simulink library "HEMERO"  (Simulink 3.00)
values from neighbouring files (symbols this model uses):
  K1 = 0.5    [ejh64.m]    (also in ejh65.m)
  K2 = 0.8    [ejh64.m]    (also in ejh65.m)
  x_camino = 0:0.01:10    [ejh64.m]    (also in ejh65.m)
  y_camino = x_camino.^2    [ejh64.m]    (also in ejh65.m)
undefined symbols (not defined in the file or in its folder): magnitude, nonlinear
libraries: simulink_extras x12, HEMERO x9, simulink3 x6, dspstat x4
(part 2 of 9)

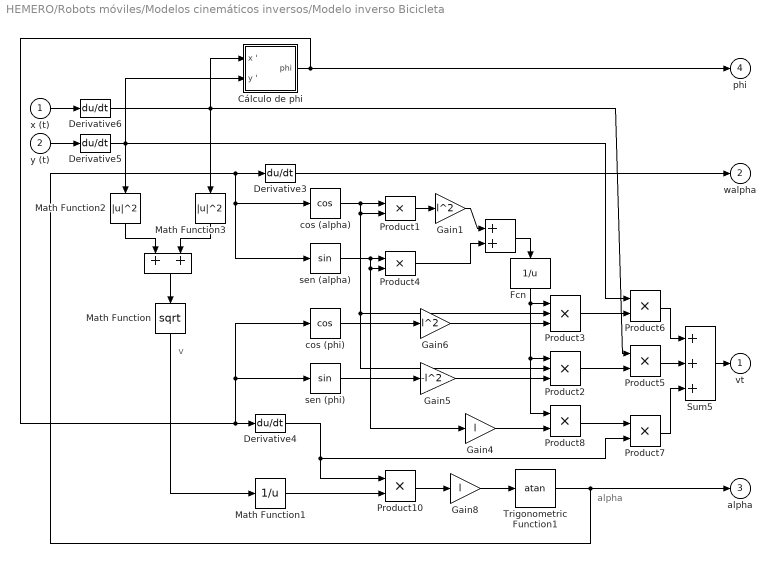
== system HEMERO/Robots móviles/Modelos cinemáticos inversos/Modelo inverso Bicicleta ==
  note: v
  note: alpha
  x (t) : Inport  Port=1  PortWidth=-1  SampleTime=-1  DataType=auto
      settings: SignalType=auto
  y (t) : Inport  Port=2  PortWidth=-1  SampleTime=-1  DataType=auto
      settings: SignalType=auto
  " " : Sum  Inputs=++  SaturateOnIntegerOverflow=on
  "  " : Sum  Orientation=down  Inputs=++  SaturateOnIntegerOverflow=on
  Cálculo de phi : Subsystem
  Derivative{3..6} (4 alike) : Derivative
  Fcn : Fcn  Orientation=down  Expr=1/u
  Gain1 : Gain  Gain=l^2  SaturateOnIntegerOverflow=on
  Gain4 : Gain  Gain=l  SaturateOnIntegerOverflow=on
  Gain5 : Gain  Gain=-l^2  SaturateOnIntegerOverflow=on
  Gain6 : Gain  Gain=l^2  SaturateOnIntegerOverflow=on
  Gain8 : Gain  Gain=l  SaturateOnIntegerOverflow=on
  Math Function : Math  Orientation=down  Operator=sqrt  OutputSignalType=auto
  Math Function1 : Math  Operator=reciprocal  OutputSignalType=auto
  Math Function2 : Math  Orientation=down  Operator=magnitude^2  OutputSignalType=auto
  Math Function3 : Math  Orientation=down  Operator=magnitude^2  OutputSignalType=auto
  Product{1,4..8,10} (7 alike) : Product  Inputs=2  SaturateOnIntegerOverflow=on
  Product2 : Product  Inputs=3  SaturateOnIntegerOverflow=on
  Product3 : Product  Inputs=3  SaturateOnIntegerOverflow=on
  Sum5 : Sum  Inputs=+++  SaturateOnIntegerOverflow=on
  Trigonometric Function1 : Trigonometry  Operator=atan  OutputSignalType=auto
  cos (alpha) : Trigonometry  Operator=cos  OutputSignalType=auto
  cos (phi) : Trigonometry  Operator=cos  OutputSignalType=auto
  sen (alpha) : Trigonometry  Operator=sin  OutputSignalType=auto
  sen (phi) : Trigonometry  Operator=sin  OutputSignalType=auto
  vt : Outport  Port=1  InitialOutput=0
  walpha : Outport  Port=2  InitialOutput=0
  alpha : Outport  Port=3  InitialOutput=0
  phi : Outport  Port=4  InitialOutput=0
  wires:
  Trigonometric Function1/1 -> alpha/1, Derivative3/1, cos (alpha)/1, sen (alpha)/1
  Cálculo de phi/1(phi) -> phi/1, cos (phi)/1, sen (phi)/1, Derivative4/1
  Math Function/1 -> Math Function1/1
  x (t)/1 -> Derivative6/1
  y (t)/1 -> Derivative5/1
  "  "/1 -> Math Function/1
  Math Function2/1 -> "  "/1
  Math Function3/1 -> "  "/2
  Derivative6/1 -> Math Function3/1, Product5/1, Cálculo de phi/1(x ')
  Derivative5/1 -> Math Function2/1, Product6/1, Cálculo de phi/2(y ')
  Gain8/1 -> Trigonometric Function1/1
  Product10/1 -> Gain8/1
  Math Function1/1 -> Product10/2
  Derivative4/1 -> Product10/1, Product7/2
  Product7/1 -> Sum5/3
  Product6/1 -> Sum5/1
  Product5/1 -> Sum5/2
  Derivative3/1 -> walpha/1
  Product8/1 -> Product7/1
  Sum5/1 -> vt/1
  Fcn/1 -> Product8/1, Product2/1, Product3/1
  Product2/1 -> Product5/2
  Gain6/1 -> Product3/3
  cos (phi)/1 -> Gain6/1
  Gain5/1 -> Product2/3
  sen (phi)/1 -> Gain5/1
  Product4/1 -> " "/2
  Product1/1 -> Gain1/1
  cos (alpha)/1 -> Product1/1, Product1/2, Product3/2, Product2/2
  sen (alpha)/1 -> Product4/2, Gain4/1, Product4/1
  " "/1 -> Fcn/1
  Gain1/1 -> " "/1
  Product3/1 -> Product6/2
  Gain4/1 -> Product8/2

== system HEMERO/Robots móviles/Modelos cinemáticos inversos/Modelo inverso Config. Síncrona ==
  x (t) : Inport  Port=1  PortWidth=-1  SampleTime=-1  DataType=auto
      settings: SignalType=auto
  y (t) : Inport  Port=2  PortWidth=-1  SampleTime=-1  DataType=auto
      settings: SignalType=auto
  Cálculo de phi : Subsystem
  Derivative : Derivative
  Derivative1 : Derivative
  Derivative2 : Derivative
  Product : Product  Inputs=2  SaturateOnIntegerOverflow=on
  Product1 : Product  Inputs=2  SaturateOnIntegerOverflow=on
  Sum : Sum  Inputs=-+  SaturateOnIntegerOverflow=on
  cos(phi) : Trigonometry  Operator=cos  OutputSignalType=auto
  sen(phi) : Trigonometry  Operator=sin  OutputSignalType=auto
  v : Outport  Port=1  InitialOutput=0
  w : Outport  Port=2  InitialOutput=0
  phi : Outport  Port=3  InitialOutput=0
  wires:
  Cálculo de phi/1(phi) -> phi/1, cos(phi)/1, Derivative2/1, sen(phi)/1
  Derivative1/1 -> Cálculo de phi/2(y '), Product1/1
  Derivative/1 -> Cálculo de phi/1(x '), Product/1
  cos(phi)/1 -> Product1/2
  sen(phi)/1 -> Product/2
  y (t)/1 -> Derivative1/1
  x (t)/1 -> Derivative/1
  Sum/1 -> v/1
  Product/1 -> Sum/1
  Product1/1 -> Sum/2
  Derivative2/1 -> w/1

== system HEMERO/Robots móviles/Modelos cinemáticos inversos/Modelo inverso Guiado Diferencial ==
  x (t) : Inport  Port=1  PortWidth=-1  SampleTime=-1  DataType=auto
      settings: SignalType=auto
  y (t) : Inport  Port=2  PortWidth=-1  SampleTime=-1  DataType=auto
      settings: SignalType=auto
  Cálculo de phi : Subsystem
  Derivative : Derivative
  Derivative1 : Derivative
  Derivative2 : Derivative
  Gain : Gain  Gain=b/2  SaturateOnIntegerOverflow=on
  Gain1 : Gain  Gain=1/c  SaturateOnIntegerOverflow=on
  Gain2 : Gain  Gain=1/c  SaturateOnIntegerOverflow=on
  Product : Product  Inputs=2  SaturateOnIntegerOverflow=on
  Product1 : Product  Inputs=2  SaturateOnIntegerOverflow=on
  Sum : Sum  Inputs=-+-  SaturateOnIntegerOverflow=on
  Sum1 : Sum  Inputs=-++  SaturateOnIntegerOverflow=on
  cos(phi) : Trigonometry  Operator=cos  OutputSignalType=auto
  sen(phi) : Trigonometry  Operator=sin  OutputSignalType=auto
  wi : Outport  Port=1  InitialOutput=0
  wd : Outport  Port=2  InitialOutput=0
  phi : Outport  Port=3  InitialOutput=0
  wires:
  x (t)/1 -> Derivative/1
  y (t)/1 -> Derivative1/1
  sen(phi)/1 -> Product/2
  cos(phi)/1 -> Product1/2
  Derivative2/1 -> Gain/1
  Product/1 -> Sum/1, Sum1/1
  Product1/1 -> Sum/2, Sum1/2
  Gain/1 -> Sum/3, Sum1/3
  Sum/1 -> Gain1/1
  Sum1/1 -> Gain2/1
  Derivative/1 -> Product/1, Cálculo de phi/1(x ')
  Derivative1/1 -> Product1/1, Cálculo de phi/2(y ')
  Cálculo de phi/1(phi) -> sen(phi)/1, Derivative2/1, cos(phi)/1, phi/1
  Gain1/1 -> wi/1
  Gain2/1 -> wd/1

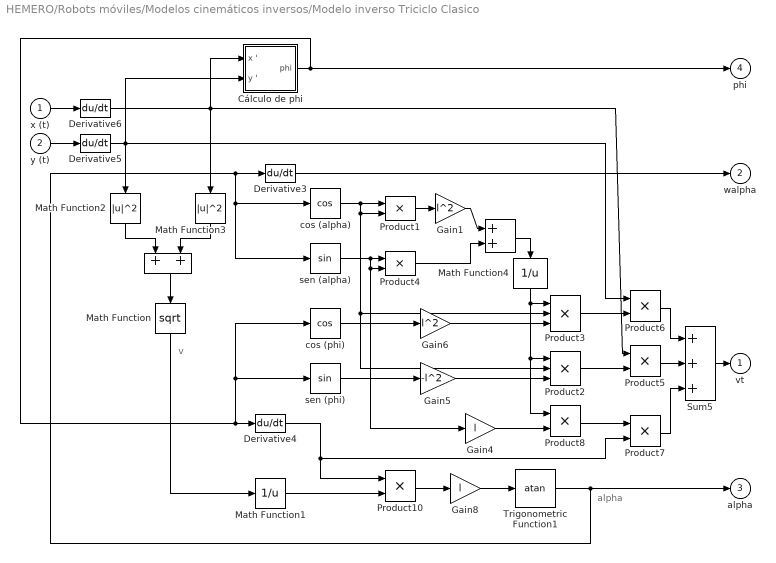
== system HEMERO/Robots móviles/Modelos cinemáticos inversos/Modelo inverso Triciclo Clasico ==
  note: alpha
  note: v
  x (t) : Inport  Port=1  PortWidth=-1  SampleTime=-1  DataType=auto
      settings: SignalType=auto
  y (t) : Inport  Port=2  PortWidth=-1  SampleTime=-1  DataType=auto
      settings: SignalType=auto
  " " : Sum  Inputs=++  SaturateOnIntegerOverflow=on
  "  " : Sum  Orientation=down  Inputs=++  SaturateOnIntegerOverflow=on
  Cálculo de phi : Subsystem
  Derivative{3..6} (4 alike) : Derivative
  Gain1 : Gain  Gain=l^2  SaturateOnIntegerOverflow=on
  Gain4 : Gain  Gain=l  SaturateOnIntegerOverflow=on
  Gain5 : Gain  Gain=-l^2  SaturateOnIntegerOverflow=on
  Gain6 : Gain  Gain=l^2  SaturateOnIntegerOverflow=on
  Gain8 : Gain  Gain=l  SaturateOnIntegerOverflow=on
  Math Function : Math  Orientation=down  Operator=sqrt  OutputSignalType=auto
  Math Function1 : Math  Operator=reciprocal  OutputSignalType=auto
  Math Function2 : Math  Orientation=down  Operator=magnitude^2  OutputSignalType=auto
  Math Function3 : Math  Orientation=down  Operator=magnitude^2  OutputSignalType=auto
  Math Function4 : Math  Orientation=down  Operator=reciprocal  OutputSignalType=auto
  Product{1,4..8,10} (7 alike) : Product  Inputs=2  SaturateOnIntegerOverflow=on
  Product2 : Product  Inputs=3  SaturateOnIntegerOverflow=on
  Product3 : Product  Inputs=3  SaturateOnIntegerOverflow=on
  Sum5 : Sum  Inputs=+++  SaturateOnIntegerOverflow=on
  Trigonometric Function1 : Trigonometry  Operator=atan  OutputSignalType=auto
  cos (alpha) : Trigonometry  Operator=cos  OutputSignalType=auto
  cos (phi) : Trigonometry  Operator=cos  OutputSignalType=auto
  sen (alpha) : Trigonometry  Operator=sin  OutputSignalType=auto
  sen (phi) : Trigonometry  Operator=sin  OutputSignalType=auto
  vt : Outport  Port=1  InitialOutput=0
  walpha : Outport  Port=2  InitialOutput=0
  alpha : Outport  Port=3  InitialOutput=0
  phi : Outport  Port=4  InitialOutput=0
  wires:
  Gain4/1 -> Product8/2
  Product3/1 -> Product6/2
  Gain1/1 -> " "/1
  " "/1 -> Math Function4/1
  sen (alpha)/1 -> Product4/1, Gain4/1, Product4/2
  cos (alpha)/1 -> Product2/2, Product3/2, Product1/2, Product1/1
  Product1/1 -> Gain1/1
  Product4/1 -> " "/2
  sen (phi)/1 -> Gain5/1
  Gain5/1 -> Product2/3
  cos (phi)/1 -> Gain6/1
  Gain6/1 -> Product3/3
  Product2/1 -> Product5/2
  Math Function4/1 -> Product3/1, Product2/1, Product8/1
  Sum5/1 -> vt/1
  Product8/1 -> Product7/1
  Derivative3/1 -> walpha/1
  Product5/1 -> Sum5/2
  Product6/1 -> Sum5/1
  Product7/1 -> Sum5/3
  Derivative4/1 -> Product7/2, Product10/1
  Math Function1/1 -> Product10/2
  Product10/1 -> Gain8/1
  Gain8/1 -> Trigonometric Function1/1
  Derivative5/1 -> Cálculo de phi/2(y '), Product6/1, Math Function2/1
  Derivative6/1 -> Cálculo de phi/1(x '), Product5/1, Math Function3/1
  Math Function3/1 -> "  "/2
  Math Function2/1 -> "  "/1
  "  "/1 -> Math Function/1
  y (t)/1 -> Derivative5/1
  x (t)/1 -> Derivative6/1
  Math Function/1 -> Math Function1/1
  Cálculo de phi/1(phi) -> Derivative4/1, sen (phi)/1, cos (phi)/1, phi/1
  Trigonometric Function1/1 -> sen (alpha)/1, cos (alpha)/1, Derivative3/1, alpha/1

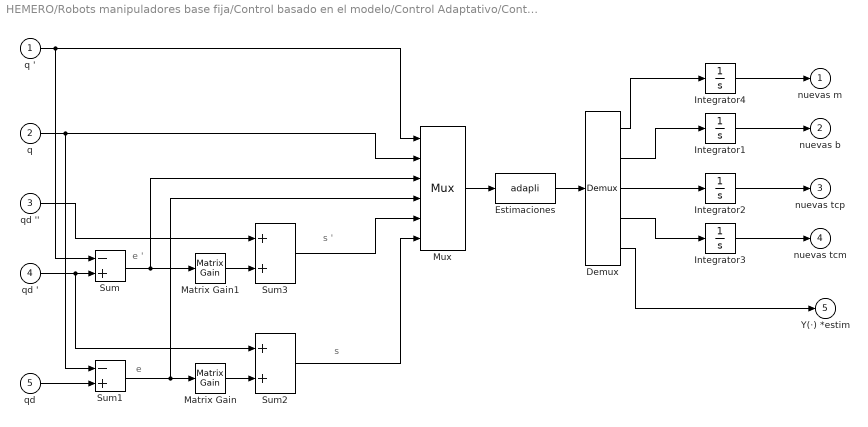
== system HEMERO/Robots manipuladores base fija/Control basado en el modelo/Control Adaptativo/Control de inercia adaptativo ==
  note: e
  note: e '
  note: s
  note: s '
  q ' : Inport  Port=1  PortWidth=-1  SampleTime=-1  DataType=auto
      settings: SignalType=auto
  q : Inport  Port=2  PortWidth=-1  SampleTime=-1  DataType=auto
      settings: SignalType=auto
  qd '' : Inport  Port=3  PortWidth=-1  SampleTime=-1  DataType=auto
      settings: SignalType=auto
  qd ' : Inport  Port=4  PortWidth=-1  SampleTime=-1  DataType=auto
      settings: SignalType=auto
  qd : Inport  Port=5  PortWidth=-1  SampleTime=-1  DataType=auto
      settings: SignalType=auto
  Demux : Demux  Outputs=5
  Estimaciones : S-Function  FunctionName=adapli  Parameters=dyn, gamma, a, grav  PortCounts=[]  SFunctionModules=''
  Integrator1 : Integrator  ExternalReset=none  InitialConditionSource=internal  InitialCondition=b_inicial(:)  LimitOutput=off  UpperSaturationLimit=inf  LowerSaturationLimit=-inf  ShowSaturationPort=off  ShowStatePort=off  AbsoluteTolerance=auto
  Integrator2 : Integrator  ExternalReset=none  InitialConditionSource=internal  InitialCondition=tcp_inicial(:)  LimitOutput=off  UpperSaturationLimit=inf  LowerSaturationLimit=-inf  ShowSaturationPort=off  ShowStatePort=off  AbsoluteTolerance=auto
  Integrator3 : Integrator  ExternalReset=none  InitialConditionSource=internal  InitialCondition=tcm_inicial(:)  LimitOutput=off  UpperSaturationLimit=inf  LowerSaturationLimit=-inf  ShowSaturationPort=off  ShowStatePort=off  AbsoluteTolerance=auto
  Integrator4 : Integrator  ExternalReset=none  InitialConditionSource=internal  InitialCondition=m_inicial(:)  LimitOutput=off  UpperSaturationLimit=inf  LowerSaturationLimit=-inf  ShowSaturationPort=off  ShowStatePort=off  AbsoluteTolerance=auto
  Matrix Gain : simulink3/Math/Matrix Gain  K=a
  Matrix Gain1 : simulink3/Math/Matrix Gain  K=a
  Mux : Mux  Inputs=6
      settings: DisplayOption=none
  Sum : Sum  Inputs=-+  SaturateOnIntegerOverflow=on
  Sum1 : Sum  Inputs=-+  SaturateOnIntegerOverflow=on
  Sum2 : Sum  Inputs=++  SaturateOnIntegerOverflow=on
  Sum3 : Sum  Inputs=++  SaturateOnIntegerOverflow=on
  nuevas m : Outport  Port=1  InitialOutput=0
  nuevas b : Outport  Port=2  InitialOutput=0
  nuevas tcp : Outport  Port=3  InitialOutput=0
  nuevas tcm : Outport  Port=4  InitialOutput=0
  Y(·) *estim : Outport  Port=5  InitialOutput=0
  wires:
  q '/1 -> Mux/1, Sum/1
  q/1 -> Mux/2, Sum1/1
  Mux/1 -> Estimaciones/1
  Estimaciones/1 -> Demux/1
  Demux/2 -> Integrator1/1
  Integrator1/1 -> nuevas b/1
  Demux/3 -> Integrator2/1
  Integrator2/1 -> nuevas tcp/1
  Demux/4 -> Integrator3/1
  Integrator3/1 -> nuevas tcm/1
  qd/1 -> Sum1/2
  Matrix Gain/1 -> Sum2/2
  qd '/1 -> Sum/2, Sum2/1
  Matrix Gain1/1 -> Sum3/2
  qd ''/1 -> Sum3/1
  Sum2/1 -> Mux/6
  Sum3/1 -> Mux/5
  Sum/1 -> Matrix Gain1/1, Mux/3
  Sum1/1 -> Matrix Gain/1, Mux/4
  Demux/5 -> Y(·) *estim/1
  Demux/1 -> Integrator4/1
  Integrator4/1 -> nuevas m/1

== system HEMERO/Robots manipuladores base fija/Control basado en el modelo/Control Adaptativo/Ejemplos ==
  Ejemplo H.5.5 : Subsystem

== system HEMERO/Robots manipuladores base fija/Control basado en el modelo/Control Adaptativo/Inversa de la matriz de masas ==
  q : Inport  Port=1  PortWidth=-1  SampleTime=-1  DataType=auto
      settings: SignalType=auto
  In : Inport  Port=2  PortWidth=-1  SampleTime=-1  DataType=auto
      settings: SignalType=auto
  nuevas m : Inport  Port=3  PortWidth=-1  SampleTime=-1  DataType=auto
      settings: SignalType=auto
  Masas : S-Function  FunctionName=esminv  Parameters=dyn  PortCounts=[]  SFunctionModules=''
  Mux : Mux  Inputs=3
      settings: DisplayOption=none
  M(q)^(-1) · In : Outport  Port=1  InitialOutput=0
  wires:
  q/1 -> Mux/1
  In/1 -> Mux/2
  nuevas m/1 -> Mux/3
  Mux/1 -> Masas/1
  Masas/1 -> M(q)^(-1) · In/1

== system HEMERO/Robots manipuladores base fija/Control basado en el modelo/Control Adaptativo/Modelo de fricciones ==
  q' : Inport  Port=1  PortWidth=-1  SampleTime=-1  DataType=auto
      settings: SignalType=auto
  nuevas b : Inport  Port=2  PortWidth=-1  SampleTime=-1  DataType=auto
      settings: SignalType=auto
  nuevas tcp : Inport  Port=3  PortWidth=-1  SampleTime=-1  DataType=auto
      settings: SignalType=auto
  nuevas tcm : Inport  Port=4  PortWidth=-1  SampleTime=-1  DataType=auto
      settings: SignalType=auto
  Fricciones : S-Function  FunctionName=esfriction  Parameters=G,b,tcp,tcm  PortCounts=[]  SFunctionModules=''
  Mux : Mux  Inputs=4
      settings: DisplayOption=none
  tau_f : Outport  Port=1  InitialOutput=0
  wires:
  Mux/1 -> Fricciones/1
  q'/1 -> Mux/1
  nuevas b/1 -> Mux/2
  nuevas tcp/1 -> Mux/3
  nuevas tcm/1 -> Mux/4
  Fricciones/1 -> tau_f/1

== system HEMERO/Robots manipuladores base fija/Control basado en el modelo/Control Adaptativo/Término Vm de Coriolis ==
  q : Inport  Port=1  PortWidth=-1  SampleTime=-1  DataType=auto
      settings: SignalType=auto
  q ' : Inport  Port=2  PortWidth=-1  SampleTime=-1  DataType=auto
      settings: SignalType=auto
  In : Inport  Port=3  PortWidth=-1  SampleTime=-1  DataType=auto
      settings: SignalType=auto
  nuevas m : Inport  Port=4  PortWidth=-1  SampleTime=-1  DataType=auto
      settings: SignalType=auto
  "  " : S-Function  FunctionName=esvmcorioli  Parameters=dyn  PortCounts=[]  SFunctionModules=''
  Mux : Mux  Inputs=4
      settings: DisplayOption=none
  Vm (q,q')·In : Outport  Port=1  InitialOutput=0
  wires:
  q '/1 -> Mux/2
  q/1 -> Mux/1
  In/1 -> Mux/3
  Mux/1 -> "  "/1
  "  "/1 -> Vm (q,q')·In/1
  nuevas m/1 -> Mux/4

== system HEMERO/Robots manipuladores base fija/Control basado en el modelo/Control Adaptativo/Término de la matriz de masas ==
  q : Inport  Port=1  PortWidth=-1  SampleTime=-1  DataType=auto
      settings: SignalType=auto
  In : Inport  Port=2  PortWidth=-1  SampleTime=-1  DataType=auto
      settings: SignalType=auto
  nuevas m : Inport  Port=3  PortWidth=-1  SampleTime=-1  DataType=auto
      settings: SignalType=auto
  Masas : S-Function  FunctionName=esinertia  Parameters=dyn  PortCounts=[]  SFunctionModules=''
  Mux : Mux  Inputs=3
      settings: DisplayOption=none
  M (q)·In : Outport  Port=1  InitialOutput=0
  wires:
  In/1 -> Mux/2
  q/1 -> Mux/1
  Mux/1 -> Masas/1
  Masas/1 -> M (q)·In/1
  nuevas m/1 -> Mux/3

== system HEMERO/Robots manipuladores base fija/Control basado en el modelo/Control Adaptativo/Términos gravitatorios ==
  q : Inport  Port=1  PortWidth=-1  SampleTime=-1  DataType=auto
      settings: SignalType=auto
  nuevas m : Inport  Port=2  PortWidth=-1  SampleTime=-1  DataType=auto
      settings: SignalType=auto
  Gravedad : S-Function  FunctionName=esgravity  Parameters=dyn,grav  PortCounts=[]  SFunctionModules=''
  Mux : Mux  Inputs=2
      settings: DisplayOption=none
  G (q) : Outport  Port=1  InitialOutput=0
  wires:
  Gravedad/1 -> G (q)/1
  q/1 -> Mux/1
  nuevas m/1 -> Mux/2
  Mux/1 -> Gravedad/1

== system HEMERO/Robots manipuladores base fija/Control basado en el modelo/Control Adaptativo/Términos centrífugos y de Coriolis ==
  q : Inport  Port=1  PortWidth=-1  SampleTime=-1  DataType=auto
      settings: SignalType=auto
  q' : Inport  Port=2  PortWidth=-1  SampleTime=-1  DataType=auto
      settings: SignalType=auto
  nuevas m : Inport  Port=3  PortWidth=-1  SampleTime=-1  DataType=auto
      settings: SignalType=auto
  Centrífugos y Coriolis : S-Function  FunctionName=escoriolis  Parameters=dyn  PortCounts=[]  SFunctionModules=''
  Mux : Mux  Inputs=3
      settings: DisplayOption=none
  V (q,q') : Outport  Port=1  InitialOutput=0
  wires:
  nuevas m/1 -> Mux/3
  Mux/1 -> Centrífugos y Coriolis/1
  Centrífugos y Coriolis/1 -> V (q,q')/1
  q/1 -> Mux/1
  q'/1 -> Mux/2

== system HEMERO/Robots manipuladores base fija/Control basado en el modelo/Control con aprendizaje/Ejemplos ==
  Ejemplo H.5.1 : Subsystem

== system HEMERO/Robots manipuladores base fija/Control basado en el modelo/Control con aprendizaje/Par realimentado aprendido ==
  note: e ''
  note: e '
  note: e
  qd '' : Inport  Port=1  PortWidth=-1  SampleTime=-1  DataType=auto
      settings: SignalType=auto
  q '' : Inport  Port=2  PortWidth=-1  SampleTime=-1  DataType=auto
      settings: SignalType=auto
  qd ' : Inport  Port=3  PortWidth=-1  SampleTime=-1  DataType=auto
      settings: SignalType=auto
  q ' : Inport  Port=4  PortWidth=-1  SampleTime=-1  DataType=auto
      settings: SignalType=auto
  qd : Inport  Port=5  PortWidth=-1  SampleTime=-1  DataType=auto
      settings: SignalType=auto
  q : Inport  Port=6  PortWidth=-1  SampleTime=-1  DataType=auto
      settings: SignalType=auto
  Demux : Demux  Outputs=4
  Mux : Mux  Inputs=3
      settings: DisplayOption=none
  S-Function : S-Function  FunctionName=learn  Parameters=Kp, Kv, mu, tfinal  PortCounts=[]  SFunctionModules=''
  Sum : Sum  Inputs=+-  SaturateOnIntegerOverflow=on
  Sum1 : Sum  Inputs=+-  SaturateOnIntegerOverflow=on
  Sum2 : Sum  Inputs=+-  SaturateOnIntegerOverflow=on
  To Workspace1 : ToWorkspace  VariableName=error  SampleTime=-1  SaveFormat=Matrix
  To Workspace2 : ToWorkspace  VariableName=error_d  SampleTime=-1  SaveFormat=Matrix
  To Workspace3 : ToWorkspace  VariableName=error_dd  SampleTime=-1  SaveFormat=Matrix
  To Workspace4 : ToWorkspace  VariableName=edd  SampleTime=-1  SaveFormat=Matrix
  To Workspace5 : ToWorkspace  VariableName=dknueva  SampleTime=-1  SaveFormat=Matrix
  To Workspace6 : ToWorkspace  VariableName=ed  SampleTime=-1  SaveFormat=Matrix
  To Workspace7 : ToWorkspace  VariableName=e  SampleTime=-1  SaveFormat=Matrix
  Término de la matriz de masas estimado : Subsystem  mask(Término asociado a la matriz de masas){dyn=dyn}
      mask prompts: dyn "Matriz de parámetros cinemáticos y dinámicos:"
      mask help: Este bloque calcula el par correspondiente al término en el que aparece la matriz de masas.
  gamma (k) : Outport  Port=1
  wires:
  Mux/1 -> S-Function/1
  S-Function/1 -> Demux/1
  qd ''/1 -> Sum/1
  q ''/1 -> Sum/2
  qd '/1 -> Sum1/1
  q '/1 -> Sum1/2
  qd/1 -> Sum2/1
  Demux/1 -> Término de la matriz de masas estimado/2(In), To Workspace5/1
  Sum2/1 -> Mux/3, To Workspace7/1
  Sum1/1 -> Mux/2, To Workspace6/1
  Sum/1 -> Mux/1, To Workspace4/1
  Demux/2 -> To Workspace1/1
  Demux/3 -> To Workspace2/1
  Demux/4 -> To Workspace3/1
  q/1 -> Sum2/2, Término de la matriz de masas estimado/1(q)
  Término de la matriz de masas estimado/1(M (q)·In) -> gamma (k)/1

== system HEMERO/Robots manipuladores base fija/Control basado en el modelo/Par Computado/Control PD ==
  qd : Inport  Port=1  PortWidth=-1  SampleTime=-1  DataType=auto
      settings: SignalType=auto
  q : Inport  Port=2  PortWidth=-1  SampleTime=-1  DataType=auto
      settings: SignalType=auto
  qd' : Inport  Port=3  PortWidth=-1  SampleTime=-1  DataType=auto
      settings: SignalType=auto
  q' : Inport  Port=4  PortWidth=-1  SampleTime=-1  DataType=auto
      settings: SignalType=auto
  qd'' : Inport  Port=5  PortWidth=-1  SampleTime=-1  DataType=auto
      settings: SignalType=auto
  Kp : StateSpace  A=[]  B=[]  C=[]  D=K  X0=0  mask(Matrix Gain){@1=Kp}
      mask prompts: @1 "Gain matrix:"
      mask help: Matrix Gain.
      mask init:
      | K=@1;
      mask Help: Multiplies input vector by entered matrix to produce output vector (y=Au).
      mask Display: disp('K')
  Kv : StateSpace  A=[]  B=[]  C=[]  D=K  X0=0  mask(Matrix Gain){@1=Kv}
      mask prompts: @1 "Gain matrix:"
      mask help: Matrix Gain.
      mask init:
      | K=@1;
      mask Help: Multiplies input vector by entered matrix to produce output vector (y=Au).
      mask Display: disp('K')
  Sum : Sum  Inputs=+-  SaturateOnIntegerOverflow=on
  Sum1 : Sum  Inputs=+-  SaturateOnIntegerOverflow=on
  Sum2 : Sum  Inputs=+++  SaturateOnIntegerOverflow=on
  tau_r : Outport  Port=1  InitialOutput=0
  wires:
  Sum2/1 -> tau_r/1
  qd''/1 -> Sum2/3
  Kp/1 -> Sum2/1
  Kv/1 -> Sum2/2
  Sum1/1 -> Kv/1
  Sum/1 -> Kp/1
  q'/1 -> Sum1/2
  qd'/1 -> Sum1/1
  q/1 -> Sum/2
  qd/1 -> Sum/1

== system HEMERO/Robots manipuladores base fija/Control basado en el modelo/Par Computado/Control PID ==
  note: e
  note: e'
  qd : Inport  Port=1  PortWidth=-1  SampleTime=-1  DataType=auto
      settings: SignalType=auto
  q : Inport  Port=2  PortWidth=-1  SampleTime=-1  DataType=auto
      settings: SignalType=auto
  qd' : Inport  Port=3  PortWidth=-1  SampleTime=-1  DataType=auto
      settings: SignalType=auto
  q' : Inport  Port=4  PortWidth=-1  SampleTime=-1  DataType=auto
      settings: SignalType=auto
  qd'' : Inport  Port=5  PortWidth=-1  SampleTime=-1  DataType=auto
      settings: SignalType=auto
  Integrator : Integrator  ExternalReset=none  InitialConditionSource=internal  InitialCondition=0  LimitOutput=off  UpperSaturationLimit=inf  LowerSaturationLimit=-inf  ShowSaturationPort=off  ShowStatePort=off  AbsoluteTolerance=auto
  Ki : StateSpace  A=[]  B=[]  C=[]  D=K  X0=0  mask(Matrix Gain){@1=Ki}
      mask prompts: @1 "Gain matrix:"
      mask help: Matrix Gain.
      mask init:
      | K=@1;
      mask Help: Multiplies input vector by entered matrix to produce output vector (y=Au).
      mask Display: disp('K')
  Kp : StateSpace  A=[]  B=[]  C=[]  D=K  X0=0  mask(Matrix Gain){@1=Kp}
      mask prompts: @1 "Gain matrix:"
      mask help: Matrix Gain.
      mask init:
      | K=@1;
      mask Help: Multiplies input vector by entered matrix to produce output vector (y=Au).
      mask Display: disp('K')
  Kv : StateSpace  A=[]  B=[]  C=[]  D=K  X0=0  mask(Matrix Gain){@1=Kv}
      mask prompts: @1 "Gain matrix:"
      mask help: Matrix Gain.
      mask init:
      | K=@1;
      mask Help: Multiplies input vector by entered matrix to produce output vector (y=Au).
      mask Display: disp('K')
  Sum : Sum  Inputs=+-  SaturateOnIntegerOverflow=on
  Sum1 : Sum  Inputs=+-  SaturateOnIntegerOverflow=on
  Sum2 : Sum  Inputs=++++  SaturateOnIntegerOverflow=on
  tau_r : Outport  Port=1  InitialOutput=0
  wires:
  Sum2/1 -> tau_r/1
  Sum1/1 -> Kv/1
  q'/1 -> Sum1/2
  qd'/1 -> Sum1/1
  q/1 -> Sum/2
  qd/1 -> Sum/1
  qd''/1 -> Sum2/4
  Kv/1 -> Sum2/3
  Kp/1 -> Sum2/2
  Sum/1 -> Kp/1, Ki/1
  Ki/1 -> Integrator/1
  Integrator/1 -> Sum2/1

== system HEMERO/Robots manipuladores base fija/Control basado en el modelo/Par Computado/Ejemplos ==
  Ejemplo H.5.2 : Subsystem
  Ejemplo H.5.3 : Subsystem
  Ejemplo H.5.4 : Subsystem

== system HEMERO/Robots manipuladores base fija/Modelo Dinámico/Ejemplos/Ejemplo H.4.2 ==
  Mux : Mux  Inputs=2
      settings: DisplayOption=none
  Tiempo : Clock
      settings: DisplayTime=off  Decimation=10
  To Workspace1 : ToWorkspace  VariableName=q  SampleTime=-1  SaveFormat=Matrix
  Trayectorias articulares : Subsystem  mask(Trayectorias articulares){dyn=[0 0 0 0 0 2 3 0 0 0 0 0 0 0 0 0 1 0 0 0; 0 3 0 0 0 1 1 0 0 0 0 0 0 0 0 0 1 0 0 0], grav=[0 -9.81 0], inivel=[0 0], inipos=[0 0]}
      mask prompts: dyn "Matriz de parámetros cinemáticos y dinámicos:"; grav "Vector aceleración de la gravedad:"; inivel "Velocidades articulares iniciales:"; inipos "Posiciones articulares iniciales:"
      mask help: Se calculan las trayectorias articulares (posiciones, velocidades y aceleraciones articulares) a partir de los pares aplicados al manipulador.
  tau1 : Fcn  Expr=30+(1+exp(-u))*10*sin(u)
  tau2 : Fcn  Expr=10+10*cos(u)
  wires:
  Mux/1 -> Trayectorias articulares/1(tau)
  Trayectorias articulares/1(q) -> To Workspace1/1
  Tiempo/1 -> tau1/1, tau2/1
  tau1/1 -> Mux/1
  tau2/1 -> Mux/2

== system HEMERO/Robots manipuladores base fija/Modelo Dinámico/Ejemplos/Ejemplo H.4.4a ==
  note: q'
  note: q''
  note: q
  Integrator : Integrator  ExternalReset=none  InitialConditionSource=internal  InitialCondition=[0;0;0]  LimitOutput=off  UpperSaturationLimit=inf  LowerSaturationLimit=-inf  ShowSaturationPort=off  ShowStatePort=off  AbsoluteTolerance=auto
  Integrator1 : Integrator  ExternalReset=none  InitialConditionSource=internal  InitialCondition=[-pi/2; 0; 0]  LimitOutput=off  UpperSaturationLimit=inf  LowerSaturationLimit=-inf  ShowSaturationPort=off  ShowStatePort=off  AbsoluteTolerance=auto
  Inversa de la matriz de masas : Subsystem  mask(Término de Coriolis){dyn=[0 0 0 0 0 4.7 0.8 0 0 0 0 0 0 0 0 0 1 0 0 0;0 0.8 0 0 0 2.6 0.8 0 0 0 0 0 0 0 0 0 1 0 0 0;0 0.8 0 0 0 1.1 0 0 0 0.05 0.1 0.1 0 0 0 0 1 0 0 0]}
      mask prompts: dyn "Matriz de parámetros dinámicos:"
      mask help: Este bloque devuelve el par correspondiente al término de Coriolis.
      mask Help: A este bloque hay que darle tres parámetros: 1) La matriz de parámetros dinámicos del manipulador de acuerdo con el formato que se explica en la sección "dyn" del Apéndice, 2) Un vector columna correspondiente a la aceleración de la gravedad, y 3) Un vector columna correspondiente a las fuerzas externas.
  Sum : Sum  Inputs=+--  SaturateOnIntegerOverflow=on
  To Workspace : ToWorkspace  VariableName=q  SampleTime=-1  SaveFormat=Matrix
  Términos gravitatorios : Subsystem  mask(Término gravitatorio){dyn=[0 0 0 0 0 4.7 0.8 0 0 0 0 0 0 0 0 0 1 0 0 0;0 0.8 0 0 0 2.6 0.8 0 0 0 0 0 0 0 0 0 1 0 0 0;0 0.8 0 0 0 1.1 0 0 0 0.05 0.1 0.1 0 0 0 0 1 0 0 0], grav=[0 -9.8 0]}
      mask prompts: dyn "Matriz de parámetros cinemáticos y dinámicos:"; grav "Vector aceleración de la gravedad:"
      mask help: Este bloque calcula el par correspondiente al término gravitatorio.
  Términos centrífugos y de Coriolis : Subsystem  mask(Términos centrífugos y de Coriolis){dyn=[0 0 0 0 0 4.7 0.8 0 0 0 0 0 0 0 0 0 1 0 0 0;0 0.8 0 0 0 2.6 0.8 0 0 0 0 0 0 0 0 0 1 0 0 0;0 0.8 0 0 0 1.1 0 0 0 0.05 0.1 0.1 0 0 0 0 1 0 0 0]}
      mask prompts: dyn "Matriz de parámetros cinemáticos y dinámicos:"
      mask help: Este bloque calcula el par correspondiente a los términos centrífugos y de Coriolis.
  q : Display
      settings: Format=short
  tau : Constant  Value=[0;0;0]
  wires:
  Términos centrífugos y de Coriolis/1(V (q,q')) -> Sum/2
  Sum/1 -> Inversa de la matriz de masas/2(In)
  Inversa de la matriz de masas/1(M(q)^(-1) · In) -> Integrator/1
  Integrator/1 -> Integrator1/1, Términos centrífugos y de Coriolis/2(q')
  Integrator1/1 -> Inversa de la matriz de masas/1(q), To Workspace/1, Términos centrífugos y de Coriolis/1(q), Términos gravitatorios/1(q), q/1
  Términos gravitatorios/1(G (q)) -> Sum/3
  tau/1 -> Sum/1

== system HEMERO/Robots manipuladores base fija/Modelo Dinámico/Ejemplos/Ejemplo H.4.4b ==
  note: q'
  note: q''
  note: q
  Integrator : Integrator  ExternalReset=none  InitialConditionSource=internal  InitialCondition=[0;0;0]  LimitOutput=off  UpperSaturationLimit=inf  LowerSaturationLimit=-inf  ShowSaturationPort=off  ShowStatePort=off  AbsoluteTolerance=auto
  Integrator1 : Integrator  ExternalReset=none  InitialConditionSource=internal  InitialCondition=[pi/6; pi/6; pi/18]  LimitOutput=off  UpperSaturationLimit=inf  LowerSaturationLimit=-inf  ShowSaturationPort=off  ShowStatePort=off  AbsoluteTolerance=auto
  Inversa de la matriz de masas : Subsystem  mask(Término de Coriolis){dyn=[0 0 0 0 0 4.7 0.8 0 0 0 0 0 0 0 0 0 1 0 0 0;0 0.8 0 0 0 2.6 0.8 0 0 0 0 0 0 0 0 0 1 0 0 0;0 0.8 0 0 0 1.1 0 0 0 0.05 0.1 0.1 0 0 0 0 1 0 0 0]}
      mask prompts: dyn "Matriz de parámetros dinámicos:"
      mask help: Este bloque devuelve el par correspondiente al término de Coriolis.
      mask Help: A este bloque hay que darle tres parámetros: 1) La matriz de parámetros dinámicos del manipulador de acuerdo con el formato que se explica en la sección "dyn" del Apéndice, 2) Un vector columna correspondiente a la aceleración de la gravedad, y 3) Un vector columna correspondiente a las fuerzas externas.
  Sum : Sum  Inputs=+--  SaturateOnIntegerOverflow=on
  To Workspace : ToWorkspace  VariableName=q  SampleTime=-1  SaveFormat=Matrix
  Términos gravitatorios : Subsystem  mask(Término gravitatorio){dyn=[0 0 0 0 0 4.7 0.8 0 0 0 0 0 0 0 0 0 1 0 0 0;0 0.8 0 0 0 2.6 0.8 0 0 0 0 0 0 0 0 0 1 0 0 0;0 0.8 0 0 0 1.1 0 0 0 0.05 0.1 0.1 0 0 0 0 1 0 0 0], grav=[0 -9.8 0]}
      mask prompts: dyn "Matriz de parámetros cinemáticos y dinámicos:"; grav "Vector aceleración de la gravedad:"
      mask help: Este bloque calcula el par correspondiente al término gravitatorio.
  Términos centrífugos y de Coriolis : Subsystem  mask(Término de Coriolis){dyn=[0 0 0 0 0 4.7 0.8 0 0 0 0 0 0 0 0 0 1 0 0 0;0 0.8 0 0 0 2.6 0.8 0 0 0 0 0 0 0 0 0 1 0 0 0;0 0.8 0 0 0 1.1 0 0 0 0.05 0.1 0.1 0 0 0 0 1 0 0 0]}
      mask prompts: dyn "Matriz de parámetros dinámicos:"
      mask help: Este bloque devuelve el par correspondiente al término de Coriolis.
      mask Help: A este bloque hay que darle tres parámetros: 1) La matriz de parámetros dinámicos del manipulador de acuerdo con el formato que se explica en la sección "dyn" del Apéndice, 2) Un vector columna correspondiente a la aceleración de la gravedad, y 3) Un vector columna correspondiente a las fuerzas externas.
  q : Display
      settings: Format=short
  tau : Constant  Value=[0;0;0]
  wires:
  Términos centrífugos y de Coriolis/1(V (q,q')) -> Sum/2
  Sum/1 -> Inversa de la matriz de masas/2(In)
  Inversa de la matriz de masas/1(M(q)^(-1) · In) -> Integrator/1
  Integrator/1 -> Integrator1/1, Términos centrífugos y de Coriolis/2(q')
  Integrator1/1 -> Inversa de la matriz de masas/1(q), To Workspace/1, Términos centrífugos y de Coriolis/1(q), Términos gravitatorios/1(q), q/1
  Términos gravitatorios/1(G (q)) -> Sum/3
  tau/1 -> Sum/1

== system HEMERO/Robots manipuladores base fija/Modelo Dinámico/Ejemplos/Ejemplo H.4.4c ==
  note: q'
  note: q''
  note: q
  Integrator : Integrator  ExternalReset=none  InitialConditionSource=internal  InitialCondition=[0;0;0]  LimitOutput=off  UpperSaturationLimit=inf  LowerSaturationLimit=-inf  ShowSaturationPort=off  ShowStatePort=off  AbsoluteTolerance=auto
  Integrator1 : Integrator  ExternalReset=none  InitialConditionSource=internal  InitialCondition=[pi/6;pi/6;pi/18]  LimitOutput=off  UpperSaturationLimit=inf  LowerSaturationLimit=-inf  ShowSaturationPort=off  ShowStatePort=off  AbsoluteTolerance=auto
  Inversa de la matriz de masas : Subsystem  mask(Término de Coriolis){dyn=[0 0 0 0 0 4.7 0.8 0 0 0 0 0 0 0 0 0 1 0 0 0;0 0.8 0 0 0 2.6 0.8 0 0 0 0 0 0 0 0 0 1 0 0 0;0 0.8 0 0 0 1.1 0 0 0 0.05 0.1 0.1 0 0 0 0 1 0 0 0]}
      mask prompts: dyn "Matriz de parámetros dinámicos:"
      mask help: Este bloque devuelve el par correspondiente al término de Coriolis.
      mask Help: A este bloque hay que darle tres parámetros: 1) La matriz de parámetros dinámicos del manipulador de acuerdo con el formato que se explica en la sección "dyn" del Apéndice, 2) Un vector columna correspondiente a la aceleración de la gravedad, y 3) Un vector columna correspondiente a las fuerzas externas.
  Modelo de fricciones1 : Subsystem  mask(Modelo de fricciones (viscosa y de Coriolis)){G=1, b=[5 5 5], tcp=[0 0 0], tcm=[0 0 0]}
      mask prompts: G "Factores de reducción (G):"; b "Fricciones viscosas, referidas al motor:"; tcp "Fricciones de Coulomb (rotación +), referidas al motor:"; tcm "Fricciones de Coulomb (rotación -), referidas al motor:"
      mask help:
      | Este bloque calcula el par correspondiente a la fricciones viscosa y de Coulomb. Para ello se emplea un determinado modelo para dichas fricciones:
      |            B·q' + Tc + ,  si q'>0
      |            B·q' + Tc - ,  si q'<0
      mask Display:
      | disp('B·q'' + Tc + ,  si q''>0\n')
      | disp('\nB·q'' + Tc - ,  si q''<0')
  Sum : Sum  Inputs=---+  SaturateOnIntegerOverflow=on
  To Workspace : ToWorkspace  VariableName=q  SampleTime=-1  SaveFormat=Matrix
  Términos gravitatorios1 : Subsystem  mask(Término gravitatorio){dyn=[0 0 0 0 0 4.7 0.8 0 0 0 0 0 0 0 0 0 1 0 0 0;0 0.8 0 0 0 2.6 0.8 0 0 0 0 0 0 0 0 0 1 0 0 0;0 0.8 0 0 0 1.1 0 0 0 0.05 0.1 0.1 0 0 0 0 1 0 0 0], grav=[0 -9.8 0]}
      mask prompts: dyn "Matriz de parámetros cinemáticos y dinámicos:"; grav "Vector aceleración de la gravedad:"
      mask help: Este bloque calcula el par correspondiente al término gravitatorio.
  Términos centrífugos y de Coriolis : Subsystem  mask(Término de Coriolis){dyn=[0 0 0 0 0 4.7 0.8 0 0 0 0 0 0 0 0 0 1 0 0 0;0 0.8 0 0 0 2.6 0.8 0 0 0 0 0 0 0 0 0 1 0 0 0;0 0.8 0 0 0 1.1 0 0 0 0.05 0.1 0.1 0 0 0 0 1 0 0 0]}
      mask prompts: dyn "Matriz de parámetros dinámicos:"
      mask help: Este bloque devuelve el par correspondiente al término de Coriolis.
      mask Help: A este bloque hay que darle tres parámetros: 1) La matriz de parámetros dinámicos del manipulador de acuerdo con el formato que se explica en la sección "dyn" del Apéndice, 2) Un vector columna correspondiente a la aceleración de la gravedad, y 3) Un vector columna correspondiente a las fuerzas externas.
  q : Display
      settings: Format=short
  tau : Constant  Value=[0;0;0]
  wires:
  Términos centrífugos y de Coriolis/1(V (q,q')) -> Sum/2
  Sum/1 -> Inversa de la matriz de masas/2(In)
  Inversa de la matriz de masas/1(M(q)^(-1) · In) -> Integrator/1
  Integrator/1 -> Integrator1/1, Términos centrífugos y de Coriolis/2(q'), Modelo de fricciones1/1(q')
  Integrator1/1 -> q/1, Términos centrífugos y de Coriolis/1(q), Términos gravitatorios1/1(q), To Workspace/1, Inversa de la matriz de masas/1(q)
  tau/1 -> Sum/4
  Términos gravitatorios1/1(G (q)) -> Sum/3
  Modelo de fricciones1/1(tau_f) -> Sum/1

== system HEMERO/Robots manipuladores base fija/Modelo Dinámico/Trayectorias articulares/Inversa de la matriz de masas ==
  q : Inport  Port=1  PortWidth=-1  SampleTime=-1  DataType=auto
      settings: SignalType=auto
  In : Inport  Port=2  PortWidth=-1  SampleTime=-1  DataType=auto
      settings: SignalType=auto
  Masas : S-Function  FunctionName=sminv  Parameters=dyn  PortCounts=[]  SFunctionModules=''
  Mux : Mux  Inputs=2
      settings: DisplayOption=none
  M(q)^(-1) · In : Outport  Port=1  InitialOutput=0
  wires:
  Mux/1 -> Masas/1
  q/1 -> Mux/1
  In/1 -> Mux/2
  Masas/1 -> M(q)^(-1) · In/1

== system HEMERO/Robots manipuladores base fija/Modelo Dinámico/Trayectorias articulares/Modelo de fricciones ==
  q' : Inport  Port=1  PortWidth=-1  SampleTime=-1  DataType=auto
      settings: SignalType=auto
  Fricciones : S-Function  FunctionName=sfriction  Parameters=G,b,tcp,tcm  PortCounts=[]  SFunctionModules=''
  tau_f : Outport  Port=1  InitialOutput=0
  wires:
  q'/1 -> Fricciones/1
  Fricciones/1 -> tau_f/1

== system HEMERO/Robots manipuladores base fija/Modelo Dinámico/Trayectorias articulares/Términos gravitatorios ==
  q : Inport  Port=1  PortWidth=-1  SampleTime=-1  DataType=auto
      settings: SignalType=auto
  Gravedad : S-Function  FunctionName=sgravity  Parameters=dyn,grav  PortCounts=[]  SFunctionModules=''
  G (q) : Outport  Port=1  InitialOutput=0
  wires:
  q/1 -> Gravedad/1
  Gravedad/1 -> G (q)/1

== system HEMERO/Robots manipuladores base fija/Modelo Dinámico/Trayectorias articulares/Términos centrífugos y de Coriolis ==
  q : Inport  Port=1  PortWidth=-1  SampleTime=-1  DataType=auto
      settings: SignalType=auto
  q' : Inport  Port=2  PortWidth=-1  SampleTime=-1  DataType=auto
      settings: SignalType=auto
  Centrífugos y Coriolis : S-Function  FunctionName=scoriolis  Parameters=dyn  PortCounts=[]  SFunctionModules=''
  Mux : Mux  Inputs=2
      settings: DisplayOption=none
  V (q,q') : Outport  Port=1  InitialOutput=0
  wires:
  Mux/1 -> Centrífugos y Coriolis/1
  q/1 -> Mux/1
  q'/1 -> Mux/2
  Centrífugos y Coriolis/1 -> V (q,q')/1

== system HEMERO/Robots manipuladores base móvil/Modelo Dinámico/Trayectorias articulares/Inversa de la matriz de masas ==
  q : Inport  Port=1  PortWidth=-1  SampleTime=-1  DataType=auto
      settings: SignalType=auto
  In : Inport  Port=2  PortWidth=-1  SampleTime=-1  DataType=auto
      settings: SignalType=auto
  w0 : Inport  Port=3  PortWidth=-1  SampleTime=-1  DataType=auto
      settings: SignalType=auto
  w0 ' : Inport  Port=4  PortWidth=-1  SampleTime=-1  DataType=auto
      settings: SignalType=auto
  v0 ' : Inport  Port=5  PortWidth=-1  SampleTime=-1  DataType=auto
      settings: SignalType=auto
  Masas : S-Function  FunctionName=msminv  Parameters=dyn  PortCounts=[]  SFunctionModules=''
  Mux : Mux  Inputs=5
      settings: DisplayOption=none
  M(q)^(-1) · In : Outport  Port=1  InitialOutput=0
  wires:
  w0 '/1 -> Mux/4
  v0 '/1 -> Mux/5
  w0/1 -> Mux/3
  Masas/1 -> M(q)^(-1) · In/1
  In/1 -> Mux/2
  q/1 -> Mux/1
  Mux/1 -> Masas/1

== system HEMERO/Robots manipuladores base móvil/Modelo Dinámico/Trayectorias articulares/Modelo de fricciones ==
  q' : Inport  Port=1  PortWidth=-1  SampleTime=-1  DataType=auto
      settings: SignalType=auto
  Fricciones : S-Function  FunctionName=sfriction  Parameters=G,b,tcp,tcm  PortCounts=[]  SFunctionModules=''
  tau_f : Outport  Port=1  InitialOutput=0
  wires:
  Fricciones/1 -> tau_f/1
  q'/1 -> Fricciones/1

== system HEMERO/Robots manipuladores base móvil/Modelo Dinámico/Trayectorias articulares/Términos gravitatorios ==
  q : Inport  Port=1  PortWidth=-1  SampleTime=-1  DataType=auto
      settings: SignalType=auto
  w0 : Inport  Port=2  PortWidth=-1  SampleTime=-1  DataType=auto
      settings: SignalType=auto
  w0 ' : Inport  Port=3  PortWidth=-1  SampleTime=-1  DataType=auto
      settings: SignalType=auto
  v0 ' : Inport  Port=4  PortWidth=-1  SampleTime=-1  DataType=auto
      settings: SignalType=auto
  Gravedad : S-Function  FunctionName=msgravity  Parameters=dyn,grav  PortCounts=[]  SFunctionModules=''
  Mux : Mux  Inputs=4
      settings: DisplayOption=none
  G (q) : Outport  Port=1  InitialOutput=0
  wires:
  Gravedad/1 -> G (q)/1
  Mux/1 -> Gravedad/1
  v0 '/1 -> Mux/4
  w0 '/1 -> Mux/3
  w0/1 -> Mux/2
  q/1 -> Mux/1

== system HEMERO/Robots manipuladores base móvil/Modelo Dinámico/Trayectorias articulares/Términos centrífugos y de Coriolis ==
  q : Inport  Port=1  PortWidth=-1  SampleTime=-1  DataType=auto
      settings: SignalType=auto
  q' : Inport  Port=2  PortWidth=-1  SampleTime=-1  DataType=auto
      settings: SignalType=auto
  w0 : Inport  Port=3  PortWidth=-1  SampleTime=-1  DataType=auto
      settings: SignalType=auto
  w0 ' : Inport  Port=4  PortWidth=-1  SampleTime=-1  DataType=auto
      settings: SignalType=auto
  v0 ' : Inport  Port=5  PortWidth=-1  SampleTime=-1  DataType=auto
      settings: SignalType=auto
  Centrífugos y Coriolis : S-Function  FunctionName=mscoriolis  Parameters=dyn  PortCounts=[]  SFunctionModules=''
  Mux : Mux  Inputs=5
      settings: DisplayOption=none
  V (q,q') : Outport  Port=1  InitialOutput=0
  wires:
  v0 '/1 -> Mux/5
  w0 '/1 -> Mux/4
  w0/1 -> Mux/3
  Centrífugos y Coriolis/1 -> V (q,q')/1
  q'/1 -> Mux/2
  q/1 -> Mux/1
  Mux/1 -> Centrífugos y Coriolis/1

== system HEMERO/Robots móviles/Control de robots móviles/Métodos geométricos/Pure Pursuit I ==
  x_vehículo : Inport  Port=1  PortWidth=-1  SampleTime=-1  DataType=auto
      settings: SignalType=auto
  y_vehículo : Inport  Port=2  PortWidth=-1  SampleTime=-1  DataType=auto
      settings: SignalType=auto
  phi_vehículo : Inport  Port=3  PortWidth=-1  SampleTime=-1  DataType=auto
      settings: SignalType=auto
  " " : Constant  Value=y_camino
  "  " : Constant  Value=x_camino
  Cálculo de incremento de x : Subsystem  Orientation=down
  Fcn : Fcn  Orientation=down  Expr=2/(u^2)
  Gain1 : Gain  Orientation=left  Gain=-1  SaturateOnIntegerOverflow=on
  Look-ahead1 : Constant  Orientation=down  Value=L
  Look-ahead2 : Constant  Value=L
  Mux : Mux  Inputs=5
      settings: DisplayOption=none
  Product : Product  Orientation=down  Inputs=2  SaturateOnIntegerOverflow=on
  Se calcula del índice del  punto que está a distancia L (pure_p_I.m) : MATLABFcn  MATLABFcn=pure_p_I  OutputWidth=-1  OutputSignalType=auto
  x_camino : Lookup  Orientation=down  InputValues=1:length(x_camino)  OutputValues=x_camino
  y_camino : Lookup  Orientation=down  InputValues=1:length(y_camino)  OutputValues=y_camino
  curvatura : Outport  Orientation=left  Port=1
  wires:
  phi_vehículo/1 -> Cálculo de incremento de x/5(phi_vehículo)
  Cálculo de incremento de x/1(incremento_x) -> Product/1
  Mux/1 -> Se calcula del índice del  punto que está a distancia L (pure_p_I.m)/1
  Look-ahead2/1 -> Mux/5
  y_vehículo/1 -> Cálculo de incremento de x/4(y_vehículo), Mux/4
  x_vehículo/1 -> Cálculo de incremento de x/3(x_vehículo), Mux/3
  " "/1 -> Mux/2
  "  "/1 -> Mux/1
  Product/1 -> Gain1/1
  Gain1/1 -> curvatura/1
  x_camino/1 -> Cálculo de incremento de x/1(x_ob)
  y_camino/1 -> Cálculo de incremento de x/2(y_ob)
  Se calcula del índice del  punto que está a distancia L (pure_p_I.m)/1 -> x_camino/1, y_camino/1
  Look-ahead1/1 -> Fcn/1
  Fcn/1 -> Product/2

== system HEMERO/Robots móviles/Control de robots móviles/Métodos geométricos/Pure Pursuit II ==
  x_vehículo : Inport  Port=1  PortWidth=-1  SampleTime=-1  DataType=auto
      settings: SignalType=auto
  y_vehículo : Inport  Port=2  PortWidth=-1  SampleTime=-1  DataType=auto
      settings: SignalType=auto
  phi_vehículo : Inport  Port=3  PortWidth=-1  SampleTime=-1  DataType=auto
      settings: SignalType=auto
  " " : Constant  Value=y_camino
  "  " : Constant  Value=x_camino
  Cálculo de L : Subsystem  Orientation=down
  Cálculo de incremento de x : Subsystem  Orientation=down
  Fcn : Fcn  Orientation=down  Expr=2/(u^2)
  Gain1 : Gain  Orientation=left  Gain=-1  SaturateOnIntegerOverflow=on
  Mux : Mux  Inputs=5
      settings: DisplayOption=none
  Product : Product  Orientation=down  Inputs=2  SaturateOnIntegerOverflow=on
  Se calcula del índice del  punto que está a distancia s sobre el camino desde el  punto del camino más próximo (pure_p_II.m) : MATLABFcn  MATLABFcn=pure_p_II  OutputWidth=-1  OutputSignalType=auto
  dist sobre el camino : Constant  Value=s
  x_camino : Lookup  Orientation=down  InputValues=1:length(x_camino)  OutputValues=x_camino
  y_camino : Lookup  Orientation=down  InputValues=1:length(y_camino)  OutputValues=y_camino
  curvatura : Outport  Orientation=left  Port=1
  wires:
  Se calcula del índice del  punto que está a distancia s sobre el camino desde el  punto del camino más próximo (pure_p_II.m)/1 -> y_camino/1, x_camino/1
  Gain1/1 -> curvatura/1
  Product/1 -> Gain1/1
  "  "/1 -> Mux/1
  " "/1 -> Mux/2
  x_vehículo/1 -> Mux/3, Cálculo de incremento de x/3(x_vehículo), Cálculo de L/3(x_vehículo)
  y_vehículo/1 -> Mux/4, Cálculo de incremento de x/4(y_vehículo), Cálculo de L/4(y_vehículo)
  dist sobre el camino/1 -> Mux/5
  Mux/1 -> Se calcula del índice del  punto que está a distancia s sobre el camino desde el  punto del camino más próximo (pure_p_II.m)/1
  Cálculo de incremento de x/1(incremento_x) -> Product/1
  phi_vehículo/1 -> Cálculo de incremento de x/5(phi_vehículo)
  Fcn/1 -> Product/2
  Cálculo de L/1(L) -> Fcn/1
  y_camino/1 -> Cálculo de incremento de x/2(y_ob), Cálculo de L/2(y_ob)
  x_camino/1 -> Cálculo de incremento de x/1(x_ob), Cálculo de L/1(x_ob)

== system HEMERO/Robots móviles/Control de robots móviles/Métodos geométricos/Pure Pursuit III ==
  x_vehículo : Inport  Port=1  PortWidth=-1  SampleTime=-1  DataType=auto
      settings: SignalType=auto
  y_vehículo : Inport  Port=2  PortWidth=-1  SampleTime=-1  DataType=auto
      settings: SignalType=auto
  phi_vehículo : Inport  Port=3  PortWidth=-1  SampleTime=-1  DataType=auto
      settings: SignalType=auto
  " " : Constant  Value=y_camino
  "  " : Constant  Value=x_camino
  Cálculo de L : Subsystem  Orientation=down
  Cálculo de incremento de x : Subsystem  Orientation=down
  Fcn : Fcn  Orientation=down  Expr=2/(u^2)
  Gain1 : Gain  Orientation=left  Gain=-1  SaturateOnIntegerOverflow=on
  Mux : Mux  Inputs=5
      settings: DisplayOption=none
  Product : Product  Orientation=down  Inputs=2  SaturateOnIntegerOverflow=on
  Saturation : Saturate  Orientation=down  UpperLimit=Lmax  LowerLimit=0
  Se calcula del índice del  punto que está a distancia s sobre el camino desde el  punto del camino más próximo (pure_p_II.m) : MATLABFcn  MATLABFcn=pure_p_II  OutputWidth=-1  OutputSignalType=auto
  dist sobre el camino : Constant  Value=s
  x_camino : Lookup  Orientation=down  InputValues=1:length(x_camino)  OutputValues=x_camino
  y_camino : Lookup  Orientation=down  InputValues=1:length(y_camino)  OutputValues=y_camino
  curvatura : Outport  Orientation=left  Port=1
  wires:
  x_camino/1 -> Cálculo de L/1(x_ob), Cálculo de incremento de x/1(x_ob)
  y_camino/1 -> Cálculo de L/2(y_ob), Cálculo de incremento de x/2(y_ob)
  Fcn/1 -> Product/2
  phi_vehículo/1 -> Cálculo de incremento de x/5(phi_vehículo)
  Cálculo de incremento de x/1(incremento_x) -> Product/1
  Mux/1 -> Se calcula del índice del  punto que está a distancia s sobre el camino desde el  punto del camino más próximo (pure_p_II.m)/1
  dist sobre el camino/1 -> Mux/5
  y_vehículo/1 -> Cálculo de L/4(y_vehículo), Cálculo de incremento de x/4(y_vehículo), Mux/4
  x_vehículo/1 -> Cálculo de L/3(x_vehículo), Cálculo de incremento de x/3(x_vehículo), Mux/3
  " "/1 -> Mux/2
  "  "/1 -> Mux/1
  Product/1 -> Gain1/1
  Gain1/1 -> curvatura/1
  Se calcula del índice del  punto que está a distancia s sobre el camino desde el  punto del camino más próximo (pure_p_II.m)/1 -> x_camino/1, y_camino/1
  Cálculo de L/1(L) -> Saturation/1
  Saturation/1 -> Fcn/1

== system HEMERO/Robots móviles/Control de robots móviles/Métodos basados en Teoría de Control/Seguimiento de caminos ==
  Ejemplos : Subsystem
  Seguimiento de caminos (control lineal) : Subsystem  mask(Seguimiento de caminos empleando una ley de control lineal){x_inicial=, y_inicial=, phi_inicial=, K1=, K2=, x_camino=, y_camino=}
      mask prompts: x_inicial "Coordenada x inicial del móvil:"; y_inicial "Coordenada y inicial del móvil:"; phi_inicial "Valor inicial de la orientación del móvil (rad):"; K1 "Parámetro K1:"; K2 "Parámetro K2:"; x_camino "Vector con las coordenadas x del camino:"; y_camino "Vector con las coordenadas y del camino:"
      mask help:
      | Este bloque permite simular una estrategia de control lineal para el seguimiento de caminos.
      | A la entrada se dispone de la velocidad del vehículo en cada instante y mediante los parámetros es posible introducir las coordenadas (x,y) del camino. A la salida se obtienen las coordenadas y orientación del vehículo en cada instante.
      mask init:
      | der_x = diff(x_camino);
      | der_y = diff(y_camino);
  Seguimiento de caminos (control no lineal) : Subsystem  mask(Seguimiento de caminos empleando una ley de control no lineal){x_inicial=, y_inicial=, phi_inicial=, K1=, K2=, x_camino=, y_camino=}
      mask prompts: x_inicial "Coordenada x inicial del móvil:"; y_inicial "Coordenada y inicial del móvil:"; phi_inicial "Valor inicial de la orientación del móvil (rad):"; K1 "Parámetro K1:"; K2 "Parámetro K2:"; x_camino "Vector con las coordenadas x del camino:"; y_camino "Vector con las coordenadas y del camino:"
      mask help:
      | Este bloque permite simular una estrategia de control no lineal para el seguimiento de caminos.
      | A la entrada se dispone de la velocidad del vehículo en cada instante y mediante los parámetros es posible introducir las coordenadas (x,y) del camino. A la salida se obtienen las coordenadas y orientación del vehículo en cada instante.
      mask init:
      | der_x = diff(x_camino);
      | der_y = diff(y_camino);
